simulink model "uas_sim"  (R2023a)
settings: Solver=VariableStepAuto  StartTime=0.0  StopTime=10.0  RelTol=1e-3  SampleTimeConstraint=STIndependent
values from neighbouring files (symbols this model uses):
  framePeriod_s = 1/frameRate_hz    (= 0.02)    [setup.m]
undefined symbols (not defined in the file or in its folder): Aircraft, datetime, datevec, Earth, Env, Fmu, InitCond, Telem, WGS84
libraries: aerolibconvert2 x8, simulink x8, aerolibadyn x3, aerolibasang x3, aerolibtransform2 x2, aerolibgravity2 x2, aerolibatmos2 x1, sharedutil x1, aerolibbdyn x1, shared6dof x1
(part 4 of 4)

== system uas_sim/Flight Management Unit/Vehicle Management System (VMS)/Variant Subsystem/FMU v2 Beta/Virtual to Non-Virtual Mapping1/Virtual to Non-Virtual Mapping4 ==
  Virtual : Inport
  Bus Creator : BusCreator  Inputs=4
  Bus Selector : BusSelector  OutputSignals=New Data,Healthy,Pressure [Pa],Die Temperature [C]
  Data Type Conversion : DataTypeConversion  OutDataTypeStr=boolean  SaturateOnIntegerOverflow=off  RndMeth=Floor
  Data Type Conversion1 : DataTypeConversion  OutDataTypeStr=boolean  SaturateOnIntegerOverflow=off  RndMeth=Floor
  Data Type Conversion2 : DataTypeConversion  OutDataTypeStr=single  SaturateOnIntegerOverflow=off  RndMeth=Floor
  Data Type Conversion3 : DataTypeConversion  OutDataTypeStr=single  SaturateOnIntegerOverflow=off  RndMeth=Floor
  Non-Virtual : Outport  OutDataTypeStr=Bus: PresData
  wires:
  Bus Creator/1 -> Non-Virtual/1
  Virtual/1 -> Bus Selector/1
  Bus Selector/1 -> Data Type Conversion/1  "<New Data>"
  Data Type Conversion/1 -> Bus Creator/1  "new_data"
  Bus Selector/2 -> Data Type Conversion1/1  "<Healthy>"
  Data Type Conversion1/1 -> Bus Creator/2  "healthy"
  Bus Selector/3 -> Data Type Conversion2/1  "<Pressure [Pa]>"
  Data Type Conversion2/1 -> Bus Creator/3  "pres_pa"
  Bus Selector/4 -> Data Type Conversion3/1  "<Die Temperature [C]>"
  Data Type Conversion3/1 -> Bus Creator/4  "die_temp_c"

== system uas_sim/Flight Management Unit/Vehicle Management System (VMS)/Variant Subsystem/FMU v2 Beta/Virtual to Non-Virtual Mapping1/Virtual to Non-Virtual Mapping5 ==
  Virtual : Inport
  Bus Creator : BusCreator  Inputs=4
  Bus Selector : BusSelector  OutputSignals=New Data,Healthy,Pressure [Pa],Die Temperature [C]
  Data Type Conversion : DataTypeConversion  OutDataTypeStr=boolean  SaturateOnIntegerOverflow=off  RndMeth=Floor
  Data Type Conversion1 : DataTypeConversion  OutDataTypeStr=boolean  SaturateOnIntegerOverflow=off  RndMeth=Floor
  Data Type Conversion2 : DataTypeConversion  OutDataTypeStr=single  SaturateOnIntegerOverflow=off  RndMeth=Floor
  Data Type Conversion3 : DataTypeConversion  OutDataTypeStr=single  SaturateOnIntegerOverflow=off  RndMeth=Floor
  Non-Virtual : Outport  OutDataTypeStr=Bus: PresData
  wires:
  Data Type Conversion3/1 -> Bus Creator/4  "die_temp_c"
  Bus Selector/4 -> Data Type Conversion3/1  "<Die Temperature [C]>"
  Data Type Conversion2/1 -> Bus Creator/3  "pres_pa"
  Bus Selector/3 -> Data Type Conversion2/1  "<Pressure [Pa]>"
  Data Type Conversion1/1 -> Bus Creator/2  "healthy"
  Bus Selector/2 -> Data Type Conversion1/1  "<Healthy>"
  Data Type Conversion/1 -> Bus Creator/1  "new_data"
  Bus Selector/1 -> Data Type Conversion/1  "<New Data>"
  Virtual/1 -> Bus Selector/1
  Bus Creator/1 -> Non-Virtual/1

== system uas_sim/Flight Management Unit/Vehicle Management System (VMS)/Variant Subsystem/FMU v2 Beta/Virtual to Non-Virtual Mapping1/Virtual to Non-Virtual Mapping6 ==
  Virtual : Inport
  Bus Creator : BusCreator  Inputs=1
  Bus Selector : BusSelector  OutputSignals=Voltages
  Data Type Conversion2 : DataTypeConversion  OutDataTypeStr=single  SaturateOnIntegerOverflow=off  RndMeth=Floor
  Non-Virtual : Outport  OutDataTypeStr=Bus: AdcData
  wires:
  Bus Creator/1 -> Non-Virtual/1
  Virtual/1 -> Bus Selector/1
  Data Type Conversion2/1 -> Bus Creator/1  "volt"
  Bus Selector/1 -> Data Type Conversion2/1  "<Voltages>"

== system uas_sim/Flight Management Unit/Vehicle Management System (VMS)/Variant Subsystem/FMU v2 Beta/Virtual to Non-Virtual Mapping5/Subsystem2 ==
  Non-Virtual : Inport  OutDataTypeStr=Bus: AnalogData
  Bus Creator : BusCreator  Inputs=1
  Bus Selector : BusSelector  OutputSignals=val
  Data Type Conversion : DataTypeConversion  OutDataTypeStr=double  SaturateOnIntegerOverflow=off  RndMeth=Floor
  Virtual : Outport
  wires:
  Non-Virtual/1 -> Bus Selector/1
  Bus Creator/1 -> Virtual/1
  Data Type Conversion/1 -> Bus Creator/1  "Values"
  Bus Selector/1 -> Data Type Conversion/1  "<val>"

== system uas_sim/Flight Management Unit/Vehicle Management System (VMS)/Variant Subsystem/FMU v2 Beta/Virtual to Non-Virtual Mapping5/Subsystem3 ==
  Non-Virtual : Inport  OutDataTypeStr=Bus: PwmCmd
  Bus Creator : BusCreator  Inputs=2
  Bus Selector : BusSelector  OutputSignals=cnt,cmd
  Data Type Conversion : DataTypeConversion  OutDataTypeStr=double  SaturateOnIntegerOverflow=off  RndMeth=Floor
  Data Type Conversion1 : DataTypeConversion  OutDataTypeStr=double  SaturateOnIntegerOverflow=off  RndMeth=Floor
  Virtual : Outport
  wires:
  Non-Virtual/1 -> Bus Selector/1
  Bus Selector/2 -> Data Type Conversion1/1  "<cmd>"
  Data Type Conversion1/1 -> Bus Creator/2  "Cmds"
  Data Type Conversion/1 -> Bus Creator/1  "Counts"
  Bus Selector/1 -> Data Type Conversion/1  "<cnt>"
  Bus Creator/1 -> Virtual/1

== system uas_sim/Flight Management Unit/Vehicle Management System (VMS)/Variant Subsystem/FMU v2 Beta/Virtual to Non-Virtual Mapping5/Subsystem4 ==
  Non-Virtual : Inport  OutDataTypeStr=Bus: SbusCmd
  Bus Creator : BusCreator  Inputs=4
  Bus Selector : BusSelector  OutputSignals=ch17,ch18,cnt,cmd
  Data Type Conversion{,1..3} (4 alike) : DataTypeConversion  OutDataTypeStr=double  SaturateOnIntegerOverflow=off  RndMeth=Floor
  Virtual : Outport
  wires:
  Non-Virtual/1 -> Bus Selector/1
  Bus Creator/1 -> Virtual/1
  Bus Selector/1 -> Data Type Conversion/1  "<ch17>"
  Bus Selector/2 -> Data Type Conversion1/1  "<ch18>"
  Bus Selector/3 -> Data Type Conversion2/1  "<cnt>"
  Bus Selector/4 -> Data Type Conversion3/1  "<cmd>"
  Data Type Conversion2/1 -> Bus Creator/3  "Counts"
  Data Type Conversion3/1 -> Bus Creator/4  "Cmds"
  Data Type Conversion1/1 -> Bus Creator/2  "Ch 18"
  Data Type Conversion/1 -> Bus Creator/1  "Ch 17"

== matlab function uas_sim/Vehicle/Vehicle Model/MATLAB Function ==
  data: ang input; ret output
function ret  = constrain360(ang)
%Constrain360 Converts a +/-180 value to a 0 - 360 value
ret = fmod(ang, 360);
if ret < 0
    ret = ret + 360;
end

end

== matlab function uas_sim/Flight Management Unit/Sensor Models/GNSS/Triggered Subsystem/MATLAB Function ==
  data: year input; month input; mday input; hour input; minute input; second input; gnss_week output; sim_clock input; gnss_tow output
function [gnss_week, gnss_tow] = GnssWeekAndTime(year, month, mday, hour, minute, second, sim_clock)

JAN61980 = 44244;
JAN11901 = 15385;
SEC_PER_DAY = 86400.0;

month_day = [
    0, 31, 59, 90, 120, 151, 181, 212, 243, 273, 304, 334;
    0, 31, 60, 91, 121, 152, 182, 213, 244, 274, 305, 335
];

second = second + sim_clock;
leap = (mod(year,4) == 0);
yday = month_day(leap + 1, month) + mday;
mjd = ((year - 1901) / 4) * 1461 + mod((year - 1901), 4) * 365 + yday - 1 + JAN11901;
fmjd = ((second / 60.0 + minute) / 60.0 + hour) / 24.0;
gnss_week = floor((mjd - JAN61980) / 7);
gnss_tow = ((mjd - JAN61980) - gnss_week * 7 + fmjd) * SEC_PER_DAY;

== matlab function uas_sim/Flight Management Unit/Sensor Models/GNSS/Triggered Subsystem/MATLAB Function1 ==
  data: ang input; ret output
function ret  = constrain360(ang)
%Constrain360 Converts a +/-180 value to a 0 - 360 value
ret = fmod(ang, 360);
if ret < 0
    ret = ret + 360;
end

end
